simulink model "simu_6c"  (R2015a)
settings: Solver=ode45  StartTime=0.0  StopTime=10.0  RelTol=1e-3
settings Model: Creator=Aluno-05  LastModifiedBy=Aluno-05

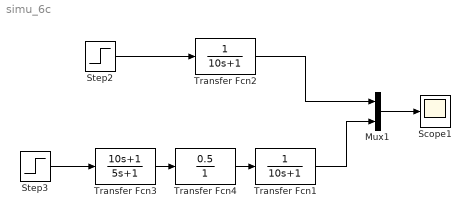
== system simu_6c ==
  Mux1 : Mux  Inputs=2
  Scope1 : Scope
  Step2 : Step  SampleTime=0
  Step3 : Step  SampleTime=0
  Transfer Fcn1 : TransferFcn  Denominator=[10 1]
  Transfer Fcn2 : TransferFcn  Denominator=[10 1]
  Transfer Fcn3 : TransferFcn  Numerator=[10 1]  Denominator=[5 1]
  Transfer Fcn4 : TransferFcn  Numerator=[0 0.5]  Denominator=[1]
  wires:
  Step2/1 -> Transfer Fcn2/1
  Transfer Fcn2/1 -> Mux1/1
  Step3/1 -> Transfer Fcn3/1
  Mux1/1 -> Scope1/1
  Transfer Fcn1/1 -> Mux1/2
  Transfer Fcn3/1 -> Transfer Fcn4/1
  Transfer Fcn4/1 -> Transfer Fcn1/1
